simulink model "IEEE30_case"  (R2024b)
settings: Solver=FixedStepAuto  StartTime=0  StopTime=5  FixedStep=1e-7  RelTol=1e-3
values from neighbouring files (symbols this model uses):
  GFL_DFIG_7_C_bus = 0.08    [IEEE30_case_parameters.m]
  GFL_DFIG_7_D_mutual = 2.500000e+3    (= 2500)    [IEEE30_case_parameters.m]
  GFL_DFIG_7_f0 = 60    [IEEE30_case_parameters.m]
  GFL_DFIG_7_gPLLi = 3200    [IEEE30_case_parameters.m]
  GFL_DFIG_7_gPLLp = 650    [IEEE30_case_parameters.m]
  GFL_DFIG_7_H_WT = 0.4    [IEEE30_case_parameters.m]
  GFL_DFIG_7_Hg = 0.8    [IEEE30_case_parameters.m]
  GFL_DFIG_7_Igq_ref = 0    [IEEE30_case_parameters.m]
  GFL_DFIG_7_Ird_ref = 704.45696    [IEEE30_case_parameters.m]
  GFL_DFIG_7_KI_V = -300000    [IEEE30_case_parameters.m]
  GFL_DFIG_7_KP_V = -1000    [IEEE30_case_parameters.m]
  GFL_DFIG_7_Ksh = 1.254300e+4    (= 12543)    [IEEE30_case_parameters.m]
  GFL_DFIG_7_Lg = 0.000483    [IEEE30_case_parameters.m]
  GFL_DFIG_7_Lm_pu = 4    [IEEE30_case_parameters.m]
  GFL_DFIG_7_N = 100    [IEEE30_case_parameters.m]
  GFL_DFIG_7_p = 2    [IEEE30_case_parameters.m]
  GFL_DFIG_7_Pitch = 0    [IEEE30_case_parameters.m]
  GFL_DFIG_7_R = 44    [IEEE30_case_parameters.m]
  GFL_DFIG_7_Rg = 2.000000e-5    (= 2e-05)    [IEEE30_case_parameters.m]
  GFL_DFIG_7_rho = 1.225    [IEEE30_case_parameters.m]
  GFL_DFIG_7_rPLLi = 4500    [IEEE30_case_parameters.m]
  GFL_DFIG_7_rPLLp = 620    [IEEE30_case_parameters.m]
  GFL_DFIG_7_Rs_pu = 0.011    [IEEE30_case_parameters.m]
  GFL_DFIG_7_Sbase = 2.000000e+6    (= 2000000)    [IEEE30_case_parameters.m]
  GFL_DFIG_7_ugq_ref = 0    [IEEE30_case_parameters.m]
  GFL_DFIG_7_usd_ref = 0    [IEEE30_case_parameters.m]
  GFL_DFIG_7_Vbase = 690    [IEEE30_case_parameters.m]
  GFL_DFIG_7_Vdc_ref = 1200    [IEEE30_case_parameters.m]
  GFL_DFIG_7_wind = 12    [IEEE30_case_parameters.m]
  GFL_DFIG_7_wm_ref = 518.184209    [IEEE30_case_parameters.m]
  SG_D_13_D = 0.01056    [IEEE30_case_parameters.m]
  SG_D_13_EnableSaturation = 0    [IEEE30_case_parameters.m]
  SG_D_13_f0 = 60    [IEEE30_case_parameters.m]
  SG_D_13_H = 7.5    [IEEE30_case_parameters.m]
  SG_D_13_K_A = 20    [IEEE30_case_parameters.m]
  SG_D_13_K_E = 1.000000e+1    (= 10)    [IEEE30_case_parameters.m]
  SG_D_13_K_F = 2.363    [IEEE30_case_parameters.m]
  SG_D_13_K_s = 0.5    [IEEE30_case_parameters.m]
  SG_D_13_R_a = 0.001088    [IEEE30_case_parameters.m]
  SG_D_13_S_A = 1    [IEEE30_case_parameters.m]
  SG_D_13_S_B = 0.103    [IEEE30_case_parameters.m]
  SG_D_13_S_N = 10.659857    [IEEE30_case_parameters.m]
  SG_D_13_SpeedPara = 200    [IEEE30_case_parameters.m]
  SG_D_13_T_0 = 0.370163    [IEEE30_case_parameters.m]
  SG_D_13_T_1 = 0.3    [IEEE30_case_parameters.m]
  SG_D_13_T_2 = 0.05    [IEEE30_case_parameters.m]
  SG_D_13_T_3 = 0.02    [IEEE30_case_parameters.m]
  SG_D_13_T_4 = 0.005    [IEEE30_case_parameters.m]
  SG_D_13_T_A = 0.02    [IEEE30_case_parameters.m]
  SG_D_13_T_dd = 8.000000e+0    (= 8)    [IEEE30_case_parameters.m]
  SG_D_13_T_ddd = 0.04    [IEEE30_case_parameters.m]
  SG_D_13_T_E = 0.314    [IEEE30_case_parameters.m]
  SG_D_13_T_F = 0.35    [IEEE30_case_parameters.m]
  SG_D_13_T_qd = 0.8    [IEEE30_case_parameters.m]
  SG_D_13_T_qdd = 0.02    [IEEE30_case_parameters.m]
  SG_D_13_T_speed = 0.1    [IEEE30_case_parameters.m]
  SG_D_13_T_w = 0.5    [IEEE30_case_parameters.m]
  SG_D_13_V_ref = 1.696619    [IEEE30_case_parameters.m]
  SG_D_13_w_ref = 376.991118    [IEEE30_case_parameters.m]
  SG_D_13_x_d = 1.9    [IEEE30_case_parameters.m]
  SG_D_13_x_dd = 0.302    [IEEE30_case_parameters.m]
  SG_D_13_x_ddd = 0.204    [IEEE30_case_parameters.m]
  SG_D_13_x_l = 0.05    [IEEE30_case_parameters.m]
  SG_D_13_x_q = 1.3    [IEEE30_case_parameters.m]
  SG_D_13_x_qd = 0.5    [IEEE30_case_parameters.m]
  SG_D_13_x_qdd = 0.3    [IEEE30_case_parameters.m]
  SG_D_1_D = 0.01056    [IEEE30_case_parameters.m]
  SG_D_1_EnableSaturation = 0    [IEEE30_case_parameters.m]
  SG_D_1_f0 = 60    [IEEE30_case_parameters.m]
  SG_D_1_H = 7.5    [IEEE30_case_parameters.m]
  SG_D_1_K_A = 20    [IEEE30_case_parameters.m]
  SG_D_1_K_E = 1.000000e+1    (= 10)    [IEEE30_case_parameters.m]
  SG_D_1_K_F = 2.363    [IEEE30_case_parameters.m]
  SG_D_1_K_s = 0.5    [IEEE30_case_parameters.m]
  SG_D_1_R_a = 0.001088    [IEEE30_case_parameters.m]
  SG_D_1_S_A = 1    [IEEE30_case_parameters.m]
  SG_D_1_S_B = 0.103    [IEEE30_case_parameters.m]
  SG_D_1_S_N = 10.659857    [IEEE30_case_parameters.m]
  SG_D_1_SpeedPara = 200    [IEEE30_case_parameters.m]
  SG_D_1_T_0 = 0.259812    [IEEE30_case_parameters.m]
  SG_D_1_T_1 = 0.3    [IEEE30_case_parameters.m]
  SG_D_1_T_2 = 0.05    [IEEE30_case_parameters.m]
  SG_D_1_T_3 = 0.02    [IEEE30_case_parameters.m]
  SG_D_1_T_4 = 0.005    [IEEE30_case_parameters.m]
  SG_D_1_T_A = 0.02    [IEEE30_case_parameters.m]
  SG_D_1_T_dd = 8.000000e+0    (= 8)    [IEEE30_case_parameters.m]
  SG_D_1_T_ddd = 0.04    [IEEE30_case_parameters.m]
  SG_D_1_T_E = 0.314    [IEEE30_case_parameters.m]
  SG_D_1_T_F = 0.35    [IEEE30_case_parameters.m]
  SG_D_1_T_qd = 0.8    [IEEE30_case_parameters.m]
  SG_D_1_T_qdd = 0.02    [IEEE30_case_parameters.m]
  SG_D_1_T_speed = 0.1    [IEEE30_case_parameters.m]
  SG_D_1_T_w = 0.5    [IEEE30_case_parameters.m]
  SG_D_1_V_ref = 1.544107    [IEEE30_case_parameters.m]
  SG_D_1_w_ref = 376.991118    [IEEE30_case_parameters.m]
  SG_D_1_x_d = 1.9    [IEEE30_case_parameters.m]
  SG_D_1_x_dd = 0.302    [IEEE30_case_parameters.m]
  SG_D_1_x_ddd = 0.204    [IEEE30_case_parameters.m]
  SG_D_1_x_l = 0.05    [IEEE30_case_parameters.m]
  SG_D_1_x_q = 1.3    [IEEE30_case_parameters.m]
  SG_D_1_x_qd = 0.5    [IEEE30_case_parameters.m]
  SG_D_1_x_qdd = 0.3    [IEEE30_case_parameters.m]
  SG_D_22_D = 0.01056    [IEEE30_case_parameters.m]
  SG_D_22_EnableSaturation = 0    [IEEE30_case_parameters.m]
  SG_D_22_f0 = 60    [IEEE30_case_parameters.m]
  SG_D_22_H = 7.5    [IEEE30_case_parameters.m]
  SG_D_22_K_A = 20    [IEEE30_case_parameters.m]
  SG_D_22_K_E = 1.000000e+1    (= 10)    [IEEE30_case_parameters.m]
  SG_D_22_K_F = 2.363    [IEEE30_case_parameters.m]
  SG_D_22_K_s = 0.5    [IEEE30_case_parameters.m]
  SG_D_22_R_a = 0.001088    [IEEE30_case_parameters.m]
  SG_D_22_S_A = 1    [IEEE30_case_parameters.m]
  SG_D_22_S_B = 0.103    [IEEE30_case_parameters.m]
  SG_D_22_S_N = 10.659857    [IEEE30_case_parameters.m]
  SG_D_22_SpeedPara = 200    [IEEE30_case_parameters.m]
  SG_D_22_T_0 = 0.216121    [IEEE30_case_parameters.m]
  SG_D_22_T_1 = 0.3    [IEEE30_case_parameters.m]
  SG_D_22_T_2 = 0.05    [IEEE30_case_parameters.m]
  SG_D_22_T_3 = 0.02    [IEEE30_case_parameters.m]
  SG_D_22_T_4 = 0.005    [IEEE30_case_parameters.m]
  ... (+126 more)
(part 26 of 27)

== system IEEE30_case/SG_D_27/d_V_f_SG_D_27_block ==
  note: d_V_f_SG_D_27 in IEEE30_case
      | $-\frac{V_{f,\mathrm{SG},D,27}-K_{A}\,\left(V_{\mathrm{ref}}-\sqrt{{\left(\frac{R_{a}\,\left(\frac{\psi _{\mathrm{1d},\mathrm{SG},D,27}\,\left(x_{\mathrm{dd}}-x_{\mathrm{ddd}}\right)}{x_{\mathrm{dd}}-x_{l}}-\psi _{d,\mathrm{SG},D,27}+\frac{\psi _{\mathrm{fd},\mathrm{SG},D,27}\,\left(x_{\mathrm{ddd}}-x_{l}\right)}{x_{\mathrm{dd}}-x_{l}}\right)}{x_{\mathrm{ddd}}}+\frac{\psi _{q,\mathrm{SG},D,27}\,w_{\mathrm{SG},D,27}}{2\,f_{0}\,\pi }\right)}^2+{\left(\frac{R_{a}\,\left(\psi _{q,\mathrm{SG},D,27}+\frac{\psi _{\mathrm{gq},\mathrm{SG},D,27}\,\left(x_{l}-x_{\mathrm{qdd}}\right)}{x_{l}-x_{\mathrm{qd}}}+\frac{\psi _{\mathrm{kq},\mathrm{SG},D,27}\,\left(x_{\mathrm{qd}}-x_{\mathrm{qdd}}\right)}{x_{l}-x_{\mathrm{qd}}}\right)}{x_{\mathrm{qdd}}}+\frac{\psi _{d,\mathrm{SG},D,27}\,w_{\mathrm{SG},D,27}}{2\,f_{0}\,\pi }\right)}^2}+K_{s}\,\mathrm{Px}_{3,\mathrm{SG},D,27}\right)-K_{A}\,R_{f,\mathrm{SG},D,27}+\frac{E_{\mathrm{fd},\mathrm{SG},D,27}\,K_{A}\,K_{F}}{T_{F}}}{T_{A}}$
      | Automatically generated on 2025-11-01 18:38:43 .
  State_E_fd_SG_D_27_11911 : Inport
  State_R_f_SG_D_27_2a887 : Inport  Port=2
  State_Px_3_SG_D_27_cca99 : Inport  Port=3
  State_psi_1d_SG_D_27_082ae : Inport  Port=4
  State_psi_d_SG_D_27_7c091 : Inport  Port=5
  State_psi_fd_SG_D_27_27c3c : Inport  Port=6
  State_psi_q_SG_D_27_dd61c : Inport  Port=7
  State_w_SG_D_27_ac390 : Inport  Port=8
  State_psi_gq_SG_D_27_6c126 : Inport  Port=9
  State_psi_kq_SG_D_27_28d7a : Inport  Port=10
  State_psi_q_SG_D_27_7ebac : Inport  Port=11
  State_psi_d_SG_D_27_c8afe : Inport  Port=12
  State_w_SG_D_27_f905c : Inport  Port=13
  State_V_f_SG_D_27_03782 : Inport  Port=14
  Add_0078a : Sum
  Add_11ebf : Sum
  Add_49114 : Sum
  Add_7f7d3 : Sum
  Add_94690 : Sum
  Add_95553 : Sum
  Add_a6206 : Sum
  Add_c1965 : Sum
  Add_cb711 : Sum
  Add_ec3d2 : Sum
  Add_fc045 : Sum
  Constant_-1_000a4 : Constant  Value=-1
  Constant_-1_049db : Constant  Value=-1
  Constant_-1_8f4b4 : Constant  Value=-1
  Constant_-1_d241f : Constant  Value=-1
  Constant_-1_dbd36 : Constant  Value=-1
  Constant_-1_dc108 : Constant  Value=-1
  Constant_2.0_3de53 : Constant  Value=2.0
  Constant_2.0_7e780 : Constant  Value=2.0
  Constant_2.0_cb466 : Constant  Value=2.0
  Constant_2.0_f5381 : Constant  Value=2.0
  Constant_K_A_68bea : Constant  Value=K_A
  Constant_K_A_bb3c1 : Constant  Value=K_A
  Constant_K_A_fd187 : Constant  Value=K_A
  Constant_K_F_7b9a8 : Constant  Value=K_F
  Constant_K_s_9c7f8 : Constant  Value=K_s
  Constant_R_a_99a15 : Constant  Value=R_a
  Constant_R_a_d0966 : Constant  Value=R_a
  Constant_T_A_b480d : Constant  Value=T_A
  Constant_T_F_69b79 : Constant  Value=T_F
  Constant_V_ref_b0cb6 : Constant  Value=V_ref
  Constant_f0_2b603 : Constant  Value=f0
  Constant_f0_d9137 : Constant  Value=f0
  Constant_pi_56945 : Constant  Value=pi
  Constant_pi_ffc0e : Constant  Value=pi
  Constant_x_dd_a9468 : Constant  Value=x_dd
  Constant_x_dd_b4216 : Constant  Value=x_dd
  Constant_x_dd_f5ebf : Constant  Value=x_dd
  Constant_x_ddd_02d42 : Constant  Value=x_ddd
  Constant_x_ddd_4227a : Constant  Value=x_ddd
  Constant_x_ddd_9297d : Constant  Value=x_ddd
  Constant_x_l_3070b : Constant  Value=x_l
  Constant_x_l_69625 : Constant  Value=x_l
  Constant_x_l_6af3f : Constant  Value=x_l
  Constant_x_l_6fbfe : Constant  Value=x_l
  Constant_x_l_b5281 : Constant  Value=x_l
  Constant_x_l_cfd51 : Constant  Value=x_l
  Constant_x_qd_26019 : Constant  Value=x_qd
  Constant_x_qd_2f63a : Constant  Value=x_qd
  Constant_x_qd_be1f0 : Constant  Value=x_qd
  Constant_x_qdd_5a1b7 : Constant  Value=x_qdd
  Constant_x_qdd_794bf : Constant  Value=x_qdd
  Constant_x_qdd_96938 : Constant  Value=x_qdd
  Divide_07c87 : Product  Inputs=*/
  Divide_1f6ef : Product  Inputs=*/
  Divide_445bd : Product  Inputs=*/
  Divide_51106 : Product  Inputs=*/
  Divide_60db4 : Product  Inputs=*/
  Divide_9589b : Product  Inputs=*/
  Divide_b7d65 : Product  Inputs=*/
  Divide_c1438 : Product  Inputs=*/
  Divide_ee8b4 : Product  Inputs=*/
  Divide_f9c68 : Product  Inputs=*/
  MathFunc_sqrt_eec58 : Sqrt
  Power_7f54e : Math  Operator=pow
  Power_84ab0 : Math  Operator=pow
  Product_09536 : Product
  Product_0e0d1 : Product
  Product_13110 : Product
  Product_152fc : Product
  Product_226c9 : Product
  Product_24809 : Product
  Product_2dce1 : Product
  Product_374ff : Product
  Product_3d675 : Product
  Product_4e57c : Product
  Product_4e8b3 : Product
  Product_6396f : Product
  Product_6fef3 : Product
  Product_9a636 : Product
  Product_9b4d0 : Product
  Product_9db0a : Product
  Product_a1a64 : Product
  Product_bfec4 : Product
  Product_c6a00 : Product
  Product_d307f : Product
  Product_d8d42 : Product
  Product_dc7be : Product
  Product_f2389 : Product
  Subtract_0c442 : Sum  Inputs=+-
  Subtract_134c1 : Sum  Inputs=+-
  Subtract_192bb : Sum  Inputs=+-
  Subtract_29f06 : Sum  Inputs=+-
  Subtract_5e59d : Sum  Inputs=+-
  Subtract_5eac6 : Sum  Inputs=+-
  Subtract_680e4 : Sum  Inputs=+-
  Subtract_9d8d6 : Sum  Inputs=+-
  Subtract_cad22 : Sum  Inputs=+-
  Blockout_d_V_f_SG_D_27_ad652 : Outport
  wires:
  Constant_-1_049db/1 -> Product_374ff/1
  Constant_x_qdd_96938/1 -> Add_7f7d3/2
  Subtract_0c442/1 -> Product_09536/2
  State_psi_d_SG_D_27_c8afe/1 -> Product_bfec4/1
  Constant_x_ddd_9297d/1 -> Subtract_0c442/2
  Constant_f0_d9137/1 -> Product_9a636/2
  Constant_-1_dbd36/1 -> Product_6396f/1
  Constant_pi_ffc0e/1 -> Product_9b4d0/2
  Product_6396f/1 -> Add_7f7d3/1
  Product_374ff/1 -> Add_11ebf/1
  Product_6fef3/1 -> Product_226c9/1
  Constant_x_l_cfd51/1 -> Product_6396f/2
  Constant_-1_8f4b4/1 -> Product_6fef3/1
  Constant_-1_000a4/1 -> Product_0e0d1/1
  State_psi_1d_SG_D_27_082ae/1 -> Product_0e0d1/2
  Constant_x_dd_a9468/1 -> Subtract_0c442/1
  Constant_-1_dc108/1 -> Product_a1a64/1
  Constant_x_qd_be1f0/1 -> Subtract_5e59d/1
  Constant_x_l_6af3f/1 -> Product_a1a64/2
  Add_a6206/1 -> Divide_1f6ef/2
  Constant_x_qdd_794bf/1 -> Subtract_5e59d/2
  Constant_x_l_6fbfe/1 -> Product_374ff/2
  Product_0e0d1/1 -> Product_09536/1
  Constant_2.0_f5381/1 -> Product_c6a00/1
  Constant_x_dd_f5ebf/1 -> Subtract_9d8d6/1
  Constant_pi_56945/1 -> Product_c6a00/2
  Divide_07c87/1 -> Add_fc045/1
  Constant_x_l_3070b/1 -> Subtract_9d8d6/2
  State_w_SG_D_27_ac390/1 -> Product_4e57c/2
  Subtract_192bb/1 -> Product_9db0a/2
  Constant_x_ddd_4227a/1 -> Subtract_192bb/1
  Constant_x_l_69625/1 -> Subtract_192bb/2
  State_psi_gq_SG_D_27_6c126/1 -> Product_24809/1
  Add_7f7d3/1 -> Product_24809/2
  Product_a1a64/1 -> Add_a6206/1
  MathFunc_sqrt_eec58/1 -> Subtract_680e4/2
  Product_2dce1/1 -> Divide_b7d65/1
  Constant_x_qd_2f63a/1 -> Add_a6206/2
  State_psi_kq_SG_D_27_28d7a/1 -> Product_2dce1/1
  Subtract_5e59d/1 -> Product_2dce1/2
  Divide_51106/1 -> Subtract_134c1/2
  Constant_x_qd_26019/1 -> Add_11ebf/2
  State_psi_d_SG_D_27_7c091/1 -> Add_fc045/2
  Product_09536/1 -> Divide_07c87/1
  Subtract_9d8d6/1 -> Divide_07c87/2
  Product_9db0a/1 -> Divide_51106/1
  State_psi_fd_SG_D_27_27c3c/1 -> Product_9db0a/1
  Subtract_cad22/1 -> Divide_51106/2
  Constant_x_dd_b4216/1 -> Subtract_cad22/1
  Constant_x_l_b5281/1 -> Subtract_cad22/2
  Product_24809/1 -> Divide_1f6ef/1
  Product_226c9/1 -> Divide_9589b/1
  Add_11ebf/1 -> Divide_b7d65/2
  Divide_1f6ef/1 -> Subtract_5eac6/1
  Divide_b7d65/1 -> Subtract_5eac6/2
  Constant_R_a_d0966/1 -> Product_6fef3/2
  Add_fc045/1 -> Subtract_134c1/1
  Constant_2.0_cb466/1 -> Product_9b4d0/1
  Subtract_5eac6/1 -> Add_49114/1
  State_psi_q_SG_D_27_7ebac/1 -> Add_49114/2
  Subtract_134c1/1 -> Product_226c9/2
  State_psi_q_SG_D_27_dd61c/1 -> Product_4e57c/1
  Product_9b4d0/1 -> Product_9a636/1
  Constant_R_a_99a15/1 -> Product_13110/1
  Add_49114/1 -> Product_13110/2
  State_w_SG_D_27_f905c/1 -> Product_bfec4/2
  Product_c6a00/1 -> Product_152fc/1
  Constant_f0_2b603/1 -> Product_152fc/2
  Constant_x_ddd_02d42/1 -> Divide_9589b/2
  Product_4e57c/1 -> Divide_60db4/1
  Product_9a636/1 -> Divide_60db4/2
  Constant_-1_d241f/1 -> Product_d307f/1
  Product_13110/1 -> Divide_f9c68/1
  Constant_x_qdd_5a1b7/1 -> Divide_f9c68/2
  Product_bfec4/1 -> Divide_445bd/1
  Product_152fc/1 -> Divide_445bd/2
  Divide_9589b/1 -> Add_94690/1
  Divide_60db4/1 -> Add_94690/2
  Divide_f9c68/1 -> Add_0078a/1
  Divide_445bd/1 -> Add_0078a/2
  State_E_fd_SG_D_27_11911/1 -> Product_d307f/2
  Add_94690/1 -> Power_7f54e/1
  Constant_2.0_7e780/1 -> Power_7f54e/2
  Add_0078a/1 -> Power_84ab0/1
  Constant_2.0_3de53/1 -> Power_84ab0/2
  Product_d307f/1 -> Product_d8d42/1
  Constant_K_A_bb3c1/1 -> Product_d8d42/2
  Constant_K_s_9c7f8/1 -> Product_dc7be/1
  State_Px_3_SG_D_27_cca99/1 -> Product_dc7be/2
  Power_7f54e/1 -> Add_cb711/1
  Power_84ab0/1 -> Add_cb711/2
  Product_d8d42/1 -> Product_f2389/1
  Constant_K_F_7b9a8/1 -> Product_f2389/2
  Product_dc7be/1 -> Add_ec3d2/1
  Constant_V_ref_b0cb6/1 -> Add_ec3d2/2
  Add_cb711/1 -> MathFunc_sqrt_eec58/1
  Product_f2389/1 -> Divide_c1438/1
  Constant_T_F_69b79/1 -> Divide_c1438/2
  Constant_K_A_68bea/1 -> Product_4e8b3/1
  State_R_f_SG_D_27_2a887/1 -> Product_4e8b3/2
  Add_ec3d2/1 -> Subtract_680e4/1
  Divide_c1438/1 -> Add_95553/1
  Product_4e8b3/1 -> Add_95553/2
  Constant_K_A_fd187/1 -> Product_3d675/1
  Subtract_680e4/1 -> Product_3d675/2
  Add_95553/1 -> Add_c1965/1
  Product_3d675/1 -> Add_c1965/2
  Add_c1965/1 -> Subtract_29f06/1
  State_V_f_SG_D_27_03782/1 -> Subtract_29f06/2
  Subtract_29f06/1 -> Divide_ee8b4/1
  Constant_T_A_b480d/1 -> Divide_ee8b4/2
  Divide_ee8b4/1 -> Blockout_d_V_f_SG_D_27_ad652/1

== system IEEE30_case/SG_D_27/d_psi_1d_SG_D_27_block ==
  note: d_psi_1d_SG_D_27 in IEEE30_case
      | $-\frac{\psi _{\mathrm{1d},\mathrm{SG},D,27}-\psi _{\mathrm{fd},\mathrm{SG},D,27}+\frac{\left(x_{\mathrm{dd}}-x_{l}\right)\,\left(\frac{\psi _{\mathrm{1d},\mathrm{SG},D,27}\,\left(x_{\mathrm{dd}}-x_{\mathrm{ddd}}\right)}{x_{\mathrm{dd}}-x_{l}}-\psi _{d,\mathrm{SG},D,27}+\frac{\psi _{\mathrm{fd},\mathrm{SG},D,27}\,\left(x_{\mathrm{ddd}}-x_{l}\right)}{x_{\mathrm{dd}}-x_{l}}\right)}{x_{\mathrm{ddd}}}}{T_{\mathrm{ddd}}}$
      | Automatically generated on 2025-11-01 18:38:18 .
  State_psi_1d_SG_D_27_efe98 : Inport
  State_psi_fd_SG_D_27_72b20 : Inport  Port=2
  State_psi_1d_SG_D_27_d0b37 : Inport  Port=3
  State_psi_d_SG_D_27_a8139 : Inport  Port=4
  State_psi_fd_SG_D_27_15400 : Inport  Port=5
  Add_984ac : Sum
  Add_acd11 : Sum
  Add_e0ec5 : Sum
  Constant_-1_6684c : Constant  Value=-1
  Constant_-1_d4480 : Constant  Value=-1
  Constant_T_ddd_242a5 : Constant  Value=T_ddd
  Constant_x_dd_17d37 : Constant  Value=x_dd
  Constant_x_dd_9a35f : Constant  Value=x_dd
  Constant_x_dd_b2bbb : Constant  Value=x_dd
  Constant_x_dd_dacc0 : Constant  Value=x_dd
  Constant_x_ddd_1b643 : Constant  Value=x_ddd
  Constant_x_ddd_29fd3 : Constant  Value=x_ddd
  Constant_x_ddd_4cc24 : Constant  Value=x_ddd
  Constant_x_l_274a7 : Constant  Value=x_l
  Constant_x_l_7e31f : Constant  Value=x_l
  Constant_x_l_91910 : Constant  Value=x_l
  Constant_x_l_d8697 : Constant  Value=x_l
  Divide_285f2 : Product  Inputs=*/
  Divide_554ff : Product  Inputs=*/
  Divide_6beb7 : Product  Inputs=*/
  Divide_8ca94 : Product  Inputs=*/
  Product_3b738 : Product
  Product_6cf61 : Product
  Product_94cdb : Product
  Product_b5c9b : Product
  Product_e0e6d : Product
  Subtract_5443c : Sum  Inputs=+-
  Subtract_b034b : Sum  Inputs=+-
  Subtract_ca0ec : Sum  Inputs=+-
  Subtract_d97b4 : Sum  Inputs=+-
  Subtract_f1971 : Sum  Inputs=+-
  Subtract_fd591 : Sum  Inputs=+-
  Blockout_d_psi_1d_SG_D_27_6915f : Outport
  wires:
  Constant_-1_6684c/1 -> Product_e0e6d/1
  State_psi_1d_SG_D_27_d0b37/1 -> Product_e0e6d/2
  Subtract_ca0ec/1 -> Product_6cf61/2
  Constant_x_ddd_1b643/1 -> Subtract_ca0ec/1
  Constant_x_dd_9a35f/1 -> Subtract_5443c/1
  Product_e0e6d/1 -> Product_b5c9b/1
  Subtract_f1971/1 -> Product_3b738/1
  Constant_x_dd_dacc0/1 -> Subtract_d97b4/1
  Constant_x_ddd_4cc24/1 -> Subtract_5443c/2
  Add_e0ec5/1 -> Add_acd11/1
  Subtract_5443c/1 -> Product_b5c9b/2
  Constant_x_l_274a7/1 -> Subtract_d97b4/2
  Add_acd11/1 -> Divide_8ca94/1
  Constant_x_l_7e31f/1 -> Subtract_ca0ec/2
  Product_b5c9b/1 -> Divide_554ff/1
  Subtract_d97b4/1 -> Divide_554ff/2
  Product_6cf61/1 -> Divide_285f2/1
  State_psi_fd_SG_D_27_15400/1 -> Product_6cf61/1
  Subtract_fd591/1 -> Divide_285f2/2
  Constant_x_dd_17d37/1 -> Subtract_fd591/1
  Constant_x_l_91910/1 -> Subtract_fd591/2
  Divide_554ff/1 -> Add_984ac/1
  Divide_285f2/1 -> Subtract_b034b/2
  State_psi_d_SG_D_27_a8139/1 -> Add_984ac/2
  Constant_x_dd_b2bbb/1 -> Subtract_f1971/1
  Constant_x_l_d8697/1 -> Subtract_f1971/2
  Add_984ac/1 -> Subtract_b034b/1
  Constant_-1_d4480/1 -> Product_94cdb/1
  State_psi_1d_SG_D_27_efe98/1 -> Product_94cdb/2
  Subtract_b034b/1 -> Product_3b738/2
  Product_94cdb/1 -> Add_e0ec5/1
  Product_3b738/1 -> Divide_6beb7/1
  State_psi_fd_SG_D_27_72b20/1 -> Add_e0ec5/2
  Constant_x_ddd_29fd3/1 -> Divide_6beb7/2
  Divide_6beb7/1 -> Add_acd11/2
  Constant_T_ddd_242a5/1 -> Divide_8ca94/2
  Divide_8ca94/1 -> Blockout_d_psi_1d_SG_D_27_6915f/1

== system IEEE30_case/SG_D_27/d_psi_d_SG_D_27_block ==
  note: d_psi_d_SG_D_27 in IEEE30_case
      | $2\,\pi \,f_{0}\,\left(v_{d,\mathrm{SG},D,27}\,\sin\left(\theta _{\mathrm{SG},D,27}\right)-v_{q,\mathrm{SG},D,27}\,\cos\left(\theta _{\mathrm{SG},D,27}\right)+\frac{R_{a}\,\left(\frac{\psi _{\mathrm{1d},\mathrm{SG},D,27}\,\left(x_{\mathrm{dd}}-x_{\mathrm{ddd}}\right)}{x_{\mathrm{dd}}-x_{l}}-\psi _{d,\mathrm{SG},D,27}+\frac{\psi _{\mathrm{fd},\mathrm{SG},D,27}\,\left(x_{\mathrm{ddd}}-x_{l}\right)}{x_{\mathrm{dd}}-x_{l}}\right)}{x_{\mathrm{ddd}}}+\frac{\psi _{q,\mathrm{SG},D,27}\,w_{\mathrm{SG},D,27}}{2\,f_{0}\,\pi }\right)$
      | Automatically generated on 2025-11-01 18:38:06 .
  State_psi_1d_SG_D_27_d5c1b : Inport
  State_psi_d_SG_D_27_a7f1f : Inport  Port=2
  State_psi_fd_SG_D_27_62224 : Inport  Port=3
  Input_v_d_SG_D_27_222f7 : Inport  Port=4
  State_theta_SG_D_27_17b48 : Inport  Port=5
  Input_v_q_SG_D_27_3207e : Inport  Port=6
  State_theta_SG_D_27_9f539 : Inport  Port=7
  State_psi_q_SG_D_27_a07c2 : Inport  Port=8
  State_w_SG_D_27_e9387 : Inport  Port=9
  Add_d6796 : Sum
  Add_dd900 : Sum
  Constant_-1_cafcc : Constant  Value=-1
  Constant_-2.0_1580e : Constant  Value=-2.0
  Constant_2.0_b6be6 : Constant  Value=2.0
  Constant_R_a_4194c : Constant  Value=R_a
  Constant_f0_77b52 : Constant  Value=f0
  Constant_f0_a4d71 : Constant  Value=f0
  Constant_pi_01718 : Constant  Value=pi
  Constant_pi_76666 : Constant  Value=pi
  Constant_x_dd_97fe1 : Constant  Value=x_dd
  Constant_x_dd_b2359 : Constant  Value=x_dd
  Constant_x_dd_c11b2 : Constant  Value=x_dd
  Constant_x_ddd_27033 : Constant  Value=x_ddd
  Constant_x_ddd_5a17f : Constant  Value=x_ddd
  Constant_x_ddd_f3053 : Constant  Value=x_ddd
  Constant_x_l_15a75 : Constant  Value=x_l
  Constant_x_l_b602a : Constant  Value=x_l
  Constant_x_l_bf8de : Constant  Value=x_l
  Divide_39e1c : Product  Inputs=*/
  Divide_7b2f6 : Product  Inputs=*/
  Divide_87c62 : Product  Inputs=*/
  Divide_b4afa : Product  Inputs=*/
  MathFunc_cos_0d1ba : Trigonometry  Operator=cos
  MathFunc_sin_08222 : Trigonometry
  Product_08f41 : Product
  Product_26066 : Product
  Product_58d64 : Product
  Product_71de0 : Product
  Product_745cc : Product
  Product_8936f : Product
  Product_9d16b : Product
  Product_a21c8 : Product
  Product_c5893 : Product
  Product_ee8b1 : Product
  Product_f3a5d : Product
  Product_f47ea : Product
  Subtract_062b2 : Sum  Inputs=+-
  Subtract_1848d : Sum  Inputs=+-
  Subtract_3d9d4 : Sum  Inputs=+-
  Subtract_5c54f : Sum  Inputs=+-
  Subtract_5feb8 : Sum  Inputs=+-
  Subtract_ab593 : Sum  Inputs=+-
  Subtract_bcda1 : Sum  Inputs=+-
  Blockout_d_psi_d_SG_D_27_ed15c : Outport
  wires:
  Divide_b4afa/1 -> Subtract_1848d/1
  Constant_x_l_15a75/1 -> Subtract_5feb8/2
  Constant_-1_cafcc/1 -> Product_a21c8/1
  Constant_x_dd_b2359/1 -> Subtract_5feb8/1
  State_psi_1d_SG_D_27_d5c1b/1 -> Product_a21c8/2
  Constant_x_dd_c11b2/1 -> Subtract_bcda1/1
  Product_8936f/1 -> Divide_b4afa/1
  Constant_x_ddd_f3053/1 -> Subtract_bcda1/2
  Product_a21c8/1 -> Product_71de0/1
  Subtract_bcda1/1 -> Product_71de0/2
  Product_26066/1 -> Product_c5893/1
  State_w_SG_D_27_e9387/1 -> Product_745cc/2
  Constant_x_ddd_27033/1 -> Subtract_5c54f/1
  Constant_x_l_bf8de/1 -> Subtract_5c54f/2
  Product_71de0/1 -> Divide_39e1c/1
  Subtract_5feb8/1 -> Divide_39e1c/2
  State_psi_fd_SG_D_27_62224/1 -> Product_9d16b/1
  Subtract_5c54f/1 -> Product_9d16b/2
  Constant_x_dd_97fe1/1 -> Subtract_062b2/1
  State_theta_SG_D_27_9f539/1 -> MathFunc_cos_0d1ba/1
  Constant_x_l_b602a/1 -> Subtract_062b2/2
  Divide_39e1c/1 -> Add_dd900/1
  Add_d6796/1 -> Subtract_ab593/1
  State_psi_d_SG_D_27_a7f1f/1 -> Add_dd900/2
  Constant_f0_77b52/1 -> Product_26066/2
  Product_9d16b/1 -> Divide_7b2f6/1
  Subtract_062b2/1 -> Divide_7b2f6/2
  Add_dd900/1 -> Subtract_3d9d4/1
  Constant_pi_76666/1 -> Product_08f41/2
  Divide_7b2f6/1 -> Subtract_3d9d4/2
  Constant_R_a_4194c/1 -> Product_8936f/1
  Subtract_3d9d4/1 -> Product_8936f/2
  MathFunc_sin_08222/1 -> Product_f47ea/2
  State_theta_SG_D_27_17b48/1 -> MathFunc_sin_08222/1
  Constant_x_ddd_5a17f/1 -> Divide_b4afa/2
  Product_f47ea/1 -> Subtract_1848d/2
  Input_v_d_SG_D_27_222f7/1 -> Product_f47ea/1
  Constant_2.0_b6be6/1 -> Product_ee8b1/1
  Input_v_q_SG_D_27_3207e/1 -> Product_f3a5d/1
  Constant_pi_01718/1 -> Product_ee8b1/2
  Constant_f0_a4d71/1 -> Product_58d64/2
  MathFunc_cos_0d1ba/1 -> Product_f3a5d/2
  Product_745cc/1 -> Divide_87c62/1
  State_psi_q_SG_D_27_a07c2/1 -> Product_745cc/1
  Product_ee8b1/1 -> Product_58d64/1
  Product_08f41/1 -> Product_26066/1
  Constant_-2.0_1580e/1 -> Product_08f41/1
  Subtract_1848d/1 -> Add_d6796/1
  Product_c5893/1 -> Blockout_d_psi_d_SG_D_27_ed15c/1
  Product_f3a5d/1 -> Add_d6796/2
  Product_58d64/1 -> Divide_87c62/2
  Divide_87c62/1 -> Subtract_ab593/2
  Subtract_ab593/1 -> Product_c5893/2

== system IEEE30_case/SG_D_27/d_psi_fd_SG_D_27_block ==
  note: d_psi_fd_SG_D_27 in IEEE30_case
      | $-\frac{\psi _{\mathrm{fd},\mathrm{SG},D,27}-E_{\mathrm{fd},\mathrm{SG},D,27}+\left(x_{d}-x_{\mathrm{dd}}\right)\,\left(\frac{\frac{\psi _{\mathrm{1d},\mathrm{SG},D,27}\,\left(x_{\mathrm{dd}}-x_{\mathrm{ddd}}\right)}{x_{\mathrm{dd}}-x_{l}}-\psi _{d,\mathrm{SG},D,27}+\frac{\psi _{\mathrm{fd},\mathrm{SG},D,27}\,\left(x_{\mathrm{ddd}}-x_{l}\right)}{x_{\mathrm{dd}}-x_{l}}}{x_{\mathrm{ddd}}}-\frac{\left(x_{\mathrm{dd}}-x_{\mathrm{ddd}}\right)\,\left(\psi _{\mathrm{1d},\mathrm{SG},D,27}-\psi _{\mathrm{fd},\mathrm{SG},D,27}+\frac{\left(x_{\mathrm{dd}}-x_{l}\right)\,\left(\frac{\psi _{\mathrm{1d},\mathrm{SG},D,27}\,\left(x_{\mathrm{dd}}-x_{\mathrm{ddd}}\right)}{x_{\mathrm{dd}}-x_{l}}-\psi _{d,\mathrm{SG},D,27}+\frac{\psi _{\mathrm{fd},\mathrm{SG},D,27}\,\left(x_{\mathrm{ddd}}-x_{l}\right)}{x_{\mathrm{dd}}-x_{l}}\right)}{x_{\mathrm{ddd}}}\right)}{{\left(x_{\mathrm{dd}}-x_{l}\right)}^2}\right)}{T_{\mathrm{dd}}}$
      | Automatically generated on 2025-11-01 18:38:15 .
  State_E_fd_SG_D_27_fdb39 : Inport
  State_psi_fd_SG_D_27_68608 : Inport  Port=2
  State_psi_1d_SG_D_27_49a09 : Inport  Port=3
  State_psi_fd_SG_D_27_f02f4 : Inport  Port=4
  State_psi_1d_SG_D_27_946b5 : Inport  Port=5
  State_psi_d_SG_D_27_fdc2b : Inport  Port=6
  State_psi_fd_SG_D_27_a093b : Inport  Port=7
  State_psi_1d_SG_D_27_1e075 : Inport  Port=8
  State_psi_d_SG_D_27_0dbb0 : Inport  Port=9
  State_psi_fd_SG_D_27_a19a0 : Inport  Port=10
  Add_1e41a : Sum
  Add_bd06a : Sum
  Constant_-1_21ffa : Constant  Value=-1
  Constant_-1_63aa3 : Constant  Value=-1
  Constant_-1_e3612 : Constant  Value=-1
  Constant_2.0_818b3 : Constant  Value=2.0
  Constant_T_dd_bea5b : Constant  Value=T_dd
  Constant_x_d_3b58c : Constant  Value=x_d
  Constant_x_dd_09696 : Constant  Value=x_dd
  Constant_x_dd_1b1b4 : Constant  Value=x_dd
  Constant_x_dd_25c64 : Constant  Value=x_dd
  Constant_x_dd_2ff33 : Constant  Value=x_dd
  Constant_x_dd_4eee0 : Constant  Value=x_dd
  Constant_x_dd_872b1 : Constant  Value=x_dd
  Constant_x_dd_af76d : Constant  Value=x_dd
  Constant_x_dd_c3d0e : Constant  Value=x_dd
  Constant_x_dd_d30d3 : Constant  Value=x_dd
  Constant_x_dd_e6b63 : Constant  Value=x_dd
  Constant_x_ddd_564f0 : Constant  Value=x_ddd
  Constant_x_ddd_5d383 : Constant  Value=x_ddd
  Constant_x_ddd_661df : Constant  Value=x_ddd
  Constant_x_ddd_83567 : Constant  Value=x_ddd
  Constant_x_ddd_d2b11 : Constant  Value=x_ddd
  Constant_x_ddd_e02b5 : Constant  Value=x_ddd
  Constant_x_ddd_e5c8e : Constant  Value=x_ddd
  Constant_x_l_006dc : Constant  Value=x_l
  Constant_x_l_55923 : Constant  Value=x_l
  Constant_x_l_66cda : Constant  Value=x_l
  Constant_x_l_6f0a9 : Constant  Value=x_l
  Constant_x_l_885e3 : Constant  Value=x_l
  Constant_x_l_8f97e : Constant  Value=x_l
  Constant_x_l_e099f : Constant  Value=x_l
  Constant_x_l_f0ec2 : Constant  Value=x_l
  Divide_144f3 : Product  Inputs=*/
  Divide_1806d : Product  Inputs=*/
  Divide_429a5 : Product  Inputs=*/
  Divide_913bf : Product  Inputs=*/
  Divide_a4ff9 : Product  Inputs=*/
  Divide_d5a08 : Product  Inputs=*/
  Divide_d6d78 : Product  Inputs=*/
  Divide_f412e : Product  Inputs=*/
  Power_5d24d : Math  Operator=pow
  Product_227af : Product
  Product_3f658 : Product
  Product_4814e : Product
  Product_4a1e5 : Product
  Product_6b77f : Product
  Product_72f51 : Product
  Product_7e8bc : Product
  Product_e2615 : Product
  Product_f0d1b : Product
  Product_f7d09 : Product
  Subtract_02cec : Sum  Inputs=+-
  Subtract_2b2a0 : Sum  Inputs=+-
  Subtract_32fb0 : Sum  Inputs=+-
  Subtract_48462 : Sum  Inputs=+-
  Subtract_4f864 : Sum  Inputs=+-
  Subtract_5da30 : Sum  Inputs=+-
  Subtract_5e343 : Sum  Inputs=+-
  Subtract_627ab : Sum  Inputs=+-
  Subtract_62b0c : Sum  Inputs=+-
  Subtract_769bd : Sum  Inputs=+-
  Subtract_89f08 : Sum  Inputs=+-
  Subtract_b9389 : Sum  Inputs=+-
  Subtract_d5a6b : Sum  Inputs=+-
  Subtract_d63e6 : Sum  Inputs=+-
  Subtract_dade3 : Sum  Inputs=+-
  Subtract_e3e3d : Sum  Inputs=+-
  Subtract_e647a : Sum  Inputs=+-
  Subtract_eecd2 : Sum  Inputs=+-
  Subtract_f34b3 : Sum  Inputs=+-
  Blockout_d_psi_fd_SG_D_27_836bf : Outport
  wires:
  Constant_-1_21ffa/1 -> Product_72f51/1
  State_psi_1d_SG_D_27_946b5/1 -> Product_72f51/2
  Product_72f51/1 -> Product_f7d09/1
  Constant_x_dd_09696/1 -> Subtract_627ab/1
  Subtract_627ab/1 -> Product_f7d09/2
  Constant_x_ddd_d2b11/1 -> Subtract_627ab/2
  Constant_x_dd_e6b63/1 -> Subtract_dade3/1
  Subtract_d63e6/1 -> Product_6b77f/1
  Constant_x_dd_1b1b4/1 -> Subtract_d63e6/1
  Constant_x_l_006dc/1 -> Subtract_dade3/2
  Constant_x_ddd_e5c8e/1 -> Divide_429a5/2
  Subtract_e3e3d/1 -> Product_4814e/2
  Constant_x_ddd_564f0/1 -> Subtract_e3e3d/1
  Subtract_89f08/1 -> Divide_a4ff9/2
  Constant_x_dd_25c64/1 -> Subtract_89f08/1
  Constant_x_l_885e3/1 -> Subtract_e3e3d/2
  Product_f7d09/1 -> Divide_144f3/1
  Subtract_dade3/1 -> Divide_144f3/2
  Product_4814e/1 -> Divide_a4ff9/1
  State_psi_fd_SG_D_27_a093b/1 -> Product_4814e/1
  Constant_x_l_f0ec2/1 -> Subtract_89f08/2
  Divide_144f3/1 -> Add_bd06a/1
  Subtract_eecd2/1 -> Power_5d24d/1
  Constant_x_dd_c3d0e/1 -> Subtract_eecd2/1
  State_psi_d_SG_D_27_fdc2b/1 -> Add_bd06a/2
  Constant_x_l_66cda/1 -> Subtract_d63e6/2
  Add_bd06a/1 -> Subtract_32fb0/1
  Divide_a4ff9/1 -> Subtract_32fb0/2
  Product_e2615/1 -> Product_3f658/1
  Constant_-1_63aa3/1 -> Product_e2615/1
  Product_3f658/1 -> Divide_d5a08/1
  State_psi_1d_SG_D_27_1e075/1 -> Product_e2615/2
  Subtract_b9389/1 -> Product_3f658/2
  Constant_x_dd_872b1/1 -> Subtract_b9389/1
  Divide_d5a08/1 -> Add_1e41a/1
  Constant_x_ddd_e02b5/1 -> Subtract_b9389/2
  Subtract_32fb0/1 -> Product_6b77f/2
  Subtract_f34b3/1 -> Divide_d5a08/2
  Constant_x_dd_af76d/1 -> Subtract_f34b3/1
  Constant_x_l_6f0a9/1 -> Subtract_f34b3/2
  Constant_x_ddd_5d383/1 -> Divide_1806d/2
  Product_f0d1b/1 -> Product_7e8bc/1
  Subtract_62b0c/1 -> Product_4a1e5/2
  Constant_x_ddd_83567/1 -> Subtract_62b0c/1
  Subtract_02cec/1 -> Subtract_e647a/1
  Constant_x_l_55923/1 -> Subtract_62b0c/2
  Constant_x_dd_4eee0/1 -> Subtract_48462/1
  Subtract_d5a6b/1 -> Divide_d6d78/2
  Subtract_48462/1 -> Product_f0d1b/2
  Constant_x_dd_d30d3/1 -> Subtract_d5a6b/1
  Constant_x_ddd_661df/1 -> Subtract_48462/2
  State_psi_1d_SG_D_27_49a09/1 -> Subtract_02cec/1
  State_psi_fd_SG_D_27_f02f4/1 -> Subtract_02cec/2
  Product_6b77f/1 -> Divide_429a5/1
  Product_4a1e5/1 -> Divide_d6d78/1
  State_psi_fd_SG_D_27_a19a0/1 -> Product_4a1e5/1
  Constant_x_l_e099f/1 -> Subtract_d5a6b/2
  Constant_-1_e3612/1 -> Product_f0d1b/1
  Divide_429a5/1 -> Subtract_e647a/2
  Constant_x_l_8f97e/1 -> Subtract_eecd2/2
  State_psi_d_SG_D_27_0dbb0/1 -> Add_1e41a/2
  Subtract_e647a/1 -> Product_7e8bc/2
  Constant_2.0_818b3/1 -> Power_5d24d/2
  Add_1e41a/1 -> Subtract_769bd/1
  Divide_d6d78/1 -> Subtract_769bd/2
  Product_7e8bc/1 -> Divide_913bf/1
  Power_5d24d/1 -> Divide_913bf/2
  Subtract_769bd/1 -> Divide_1806d/1
  Constant_x_d_3b58c/1 -> Subtract_5da30/1
  Constant_x_dd_2ff33/1 -> Subtract_5da30/2
  Divide_913bf/1 -> Subtract_2b2a0/1
  Divide_1806d/1 -> Subtract_2b2a0/2
  State_E_fd_SG_D_27_fdb39/1 -> Subtract_5e343/1
  State_psi_fd_SG_D_27_68608/1 -> Subtract_5e343/2
  Subtract_5da30/1 -> Product_227af/1
  Subtract_2b2a0/1 -> Product_227af/2
  Subtract_5e343/1 -> Subtract_4f864/1
  Product_227af/1 -> Subtract_4f864/2
  Subtract_4f864/1 -> Divide_f412e/1
  Constant_T_dd_bea5b/1 -> Divide_f412e/2
  Divide_f412e/1 -> Blockout_d_psi_fd_SG_D_27_836bf/1

== system IEEE30_case/SG_D_27/d_psi_gq_SG_D_27_block ==
  note: d_psi_gq_SG_D_27 in IEEE30_case
      | $-\frac{\psi _{\mathrm{gq},\mathrm{SG},D,27}+\left(x_{q}-x_{\mathrm{qd}}\right)\,\left(\frac{\psi _{q,\mathrm{SG},D,27}+\frac{\psi _{\mathrm{gq},\mathrm{SG},D,27}\,\left(x_{l}-x_{\mathrm{qdd}}\right)}{x_{l}-x_{\mathrm{qd}}}+\frac{\psi _{\mathrm{kq},\mathrm{SG},D,27}\,\left(x_{\mathrm{qd}}-x_{\mathrm{qdd}}\right)}{x_{l}-x_{\mathrm{qd}}}}{x_{\mathrm{qdd}}}+\frac{\left(x_{\mathrm{qd}}-x_{\mathrm{qdd}}\right)\,\left(\psi _{\mathrm{gq},\mathrm{SG},D,27}+\psi _{\mathrm{kq},\mathrm{SG},D,27}+\frac{\left(x_{l}-x_{\mathrm{qd}}\right)\,\left(\psi _{q,\mathrm{SG},D,27}+\frac{\psi _{\mathrm{gq},\mathrm{SG},D,27}\,\left(x_{l}-x_{\mathrm{qdd}}\right)}{x_{l}-x_{\mathrm{qd}}}+\frac{\psi _{\mathrm{kq},\mathrm{SG},D,27}\,\left(x_{\mathrm{qd}}-x_{\mathrm{qdd}}\right)}{x_{l}-x_{\mathrm{qd}}}\right)}{x_{\mathrm{qdd}}}\right)}{{\left(x_{l}-x_{\mathrm{qd}}\right)}^2}\right)}{T_{\mathrm{qd}}}$
      | Automatically generated on 2025-11-01 18:38:24 .
  State_psi_gq_SG_D_27_c3af2 : Inport
  State_psi_gq_SG_D_27_6e8f7 : Inport  Port=2
  State_psi_kq_SG_D_27_7c836 : Inport  Port=3
  State_psi_gq_SG_D_27_3e2b9 : Inport  Port=4
  State_psi_kq_SG_D_27_4dbff : Inport  Port=5
  State_psi_q_SG_D_27_a0060 : Inport  Port=6
  State_psi_gq_SG_D_27_ed82f : Inport  Port=7
  State_psi_kq_SG_D_27_09d28 : Inport  Port=8
  State_psi_q_SG_D_27_f7919 : Inport  Port=9
  Add_1e70e : Sum
  Add_48da1 : Sum
  Add_4b738 : Sum
  Add_73542 : Sum
  Add_7e406 : Sum
  Add_85f35 : Sum
  Add_9c560 : Sum
  Add_b110a : Sum
  Add_bba7d : Sum
  Add_c43b7 : Sum
  Add_c9cb5 : Sum
  Add_e5e6a : Sum
  Constant_-1_058df : Constant  Value=-1
  Constant_-1_0983a : Constant  Value=-1
  Constant_-1_14dd2 : Constant  Value=-1
  Constant_-1_14efb : Constant  Value=-1
  Constant_-1_28226 : Constant  Value=-1
  Constant_-1_3ef3e : Constant  Value=-1
  Constant_-1_4fa86 : Constant  Value=-1
  Constant_-1_6b263 : Constant  Value=-1
  Constant_-1_9d686 : Constant  Value=-1
  Constant_-1_d0f9f : Constant  Value=-1
  Constant_2.0_312bc : Constant  Value=2.0
  Constant_T_qd_feea3 : Constant  Value=T_qd
  Constant_x_l_14cc6 : Constant  Value=x_l
  Constant_x_l_1677c : Constant  Value=x_l
  Constant_x_l_54f9f : Constant  Value=x_l
  Constant_x_l_793c4 : Constant  Value=x_l
  Constant_x_l_8c285 : Constant  Value=x_l
  Constant_x_l_a146c : Constant  Value=x_l
  Constant_x_l_d0309 : Constant  Value=x_l
  Constant_x_l_f9961 : Constant  Value=x_l
  Constant_x_q_90015 : Constant  Value=x_q
  Constant_x_qd_07190 : Constant  Value=x_qd
  Constant_x_qd_20e3c : Constant  Value=x_qd
  Constant_x_qd_38946 : Constant  Value=x_qd
  Constant_x_qd_5e3be : Constant  Value=x_qd
  Constant_x_qd_b0be0 : Constant  Value=x_qd
  Constant_x_qd_b7f1f : Constant  Value=x_qd
  Constant_x_qd_c908f : Constant  Value=x_qd
  Constant_x_qd_d4f0d : Constant  Value=x_qd
  Constant_x_qd_e9b47 : Constant  Value=x_qd
  Constant_x_qd_e9e12 : Constant  Value=x_qd
  Constant_x_qdd_51bb0 : Constant  Value=x_qdd
  Constant_x_qdd_699cd : Constant  Value=x_qdd
  Constant_x_qdd_6ad97 : Constant  Value=x_qdd
  Constant_x_qdd_81391 : Constant  Value=x_qdd
  Constant_x_qdd_bfc03 : Constant  Value=x_qdd
  Constant_x_qdd_e17ca : Constant  Value=x_qdd
  Constant_x_qdd_fe73c : Constant  Value=x_qdd
  Divide_2b076 : Product  Inputs=*/
  Divide_4a76a : Product  Inputs=*/
  Divide_638f3 : Product  Inputs=*/
  Divide_647d7 : Product  Inputs=*/
  Divide_a909f : Product  Inputs=*/
  Divide_b7c1d : Product  Inputs=*/
  Divide_cbeb0 : Product  Inputs=*/
  Divide_e205d : Product  Inputs=*/
  Power_6b5ce : Math  Operator=pow
  Product_1d788 : Product
  Product_242e9 : Product
  Product_26390 : Product
  Product_3603a : Product
  Product_450c3 : Product
  Product_56ad6 : Product
  Product_57164 : Product
  Product_8ca79 : Product
  Product_994b8 : Product
  Product_996e2 : Product
  Product_9be87 : Product
  Product_a6325 : Product
  Product_b10ae : Product
  Product_bef90 : Product
  Product_c8340 : Product
  Product_c97cd : Product
  Product_fec86 : Product
  Subtract_2a6c1 : Sum  Inputs=+-
  Subtract_3ad86 : Sum  Inputs=+-
  Subtract_808bf : Sum  Inputs=+-
  Subtract_84fe7 : Sum  Inputs=+-
  Subtract_a1eb2 : Sum  Inputs=+-
  Subtract_a74ec : Sum  Inputs=+-
  Subtract_d1765 : Sum  Inputs=+-
  Subtract_ea8bb : Sum  Inputs=+-
  Blockout_d_psi_gq_SG_D_27_e3839 : Outport
  wires:
  State_psi_gq_SG_D_27_6e8f7/1 -> Add_73542/1
  Constant_x_l_1677c/1 -> Product_3603a/2
  Constant_x_l_d0309/1 -> Product_450c3/2
  Constant_-1_9d686/1 -> Product_57164/1
  Product_57164/1 -> Add_85f35/1
  Constant_x_l_793c4/1 -> Product_57164/2
  Constant_x_l_f9961/1 -> Product_26390/2
  Divide_e205d/1 -> Blockout_d_psi_gq_SG_D_27_e3839/1
  Constant_x_qd_e9e12/1 -> Subtract_d1765/1
  Constant_x_qdd_fe73c/1 -> Add_85f35/2
  Add_e5e6a/1 -> Divide_a909f/2
  Product_fec86/1 -> Divide_638f3/1
  Constant_-1_058df/1 -> Product_3603a/1
  Constant_x_qdd_51bb0/1 -> Subtract_d1765/2
  Constant_x_l_8c285/1 -> Product_9be87/2
  Constant_-1_14efb/1 -> Product_994b8/1
  Constant_x_l_a146c/1 -> Product_994b8/2
  Constant_x_l_54f9f/1 -> Product_56ad6/2
  State_psi_gq_SG_D_27_3e2b9/1 -> Product_c97cd/1
  Add_85f35/1 -> Product_c97cd/2
  Constant_x_qdd_6ad97/1 -> Subtract_2a6c1/2
  Subtract_3ad86/1 -> Product_b10ae/2
  Product_3603a/1 -> Add_c9cb5/1
  Constant_x_qd_20e3c/1 -> Add_c9cb5/2
  Subtract_2a6c1/1 -> Product_8ca79/2
  Constant_x_qd_38946/1 -> Subtract_2a6c1/1
  State_psi_kq_SG_D_27_4dbff/1 -> Product_996e2/1
  Subtract_d1765/1 -> Product_996e2/2
  Product_994b8/1 -> Add_9c560/1
  Add_1e70e/1 -> Product_c8340/2
  Constant_x_qd_d4f0d/1 -> Add_9c560/2
  Product_c97cd/1 -> Divide_b7c1d/1
  Add_c9cb5/1 -> Divide_b7c1d/2
  Product_996e2/1 -> Divide_2b076/1
  Add_9c560/1 -> Divide_2b076/2
  Product_242e9/1 -> Add_7e406/1
  Constant_-1_28226/1 -> Product_242e9/1
  Constant_x_qd_b7f1f/1 -> Add_e5e6a/2
  Constant_x_l_14cc6/1 -> Product_242e9/2
  Constant_x_qdd_699cd/1 -> Subtract_a74ec/2
  Divide_b7c1d/1 -> Subtract_a1eb2/1
  Divide_2b076/1 -> Subtract_a1eb2/2
  Product_9be87/1 -> Add_1e70e/1
  State_psi_q_SG_D_27_a0060/1 -> Add_bba7d/2
  Constant_-1_6b263/1 -> Product_9be87/1
  Constant_x_qd_07190/1 -> Add_7e406/2
  Product_a6325/1 -> Add_c43b7/1
  Constant_x_qd_c908f/1 -> Add_48da1/2
  Subtract_a1eb2/1 -> Add_bba7d/1
  Constant_x_qdd_bfc03/1 -> Add_1e70e/2
  Constant_-1_0983a/1 -> Product_1d788/1
  Product_56ad6/1 -> Add_48da1/1
  Constant_-1_4fa86/1 -> Product_56ad6/1
  Product_450c3/1 -> Add_e5e6a/1
  Add_7e406/1 -> Product_fec86/1
  Constant_-1_3ef3e/1 -> Product_450c3/1
  Add_bba7d/1 -> Product_fec86/2
  Product_c8340/1 -> Divide_cbeb0/1
  State_psi_gq_SG_D_27_ed82f/1 -> Product_c8340/1
  Product_8ca79/1 -> Divide_a909f/1
  State_psi_kq_SG_D_27_09d28/1 -> Product_8ca79/1
  Constant_x_qd_e9b47/1 -> Subtract_a74ec/1
  State_psi_kq_SG_D_27_7c836/1 -> Add_73542/2
  Constant_x_qdd_81391/1 -> Divide_638f3/2
  Constant_-1_14dd2/1 -> Product_26390/1
  Add_48da1/1 -> Divide_cbeb0/2
  Subtract_a74ec/1 -> Product_1d788/2
  Add_73542/1 -> Subtract_ea8bb/1
  Divide_638f3/1 -> Subtract_ea8bb/2
  Product_26390/1 -> Add_b110a/1
  Constant_x_qd_5e3be/1 -> Add_b110a/2
  Divide_cbeb0/1 -> Subtract_808bf/1
  State_psi_q_SG_D_27_f7919/1 -> Add_4b738/2
  Divide_a909f/1 -> Subtract_808bf/2
  Product_1d788/1 -> Product_bef90/1
  Subtract_ea8bb/1 -> Product_bef90/2
  Add_b110a/1 -> Power_6b5ce/1
  Constant_2.0_312bc/1 -> Power_6b5ce/2
  Subtract_808bf/1 -> Add_4b738/1
  Product_bef90/1 -> Divide_4a76a/1
  Power_6b5ce/1 -> Divide_4a76a/2
  Add_4b738/1 -> Divide_647d7/1
  Constant_x_qdd_e17ca/1 -> Divide_647d7/2
  Constant_x_q_90015/1 -> Subtract_84fe7/1
  Constant_x_qd_b0be0/1 -> Subtract_84fe7/2
  Divide_4a76a/1 -> Subtract_3ad86/1
  Constant_-1_d0f9f/1 -> Product_a6325/1
  Divide_647d7/1 -> Subtract_3ad86/2
  State_psi_gq_SG_D_27_c3af2/1 -> Product_a6325/2
  Subtract_84fe7/1 -> Product_b10ae/1
  Product_b10ae/1 -> Add_c43b7/2
  Add_c43b7/1 -> Divide_e205d/1
  Constant_T_qd_feea3/1 -> Divide_e205d/2

== system IEEE30_case/SG_D_27/d_psi_kq_SG_D_27_block ==
  note: d_psi_kq_SG_D_27 in IEEE30_case
      | $-\frac{\psi _{\mathrm{gq},\mathrm{SG},D,27}+\psi _{\mathrm{kq},\mathrm{SG},D,27}+\frac{\left(x_{l}-x_{\mathrm{qd}}\right)\,\left(\psi _{q,\mathrm{SG},D,27}+\frac{\psi _{\mathrm{gq},\mathrm{SG},D,27}\,\left(x_{l}-x_{\mathrm{qdd}}\right)}{x_{l}-x_{\mathrm{qd}}}+\frac{\psi _{\mathrm{kq},\mathrm{SG},D,27}\,\left(x_{\mathrm{qd}}-x_{\mathrm{qdd}}\right)}{x_{l}-x_{\mathrm{qd}}}\right)}{x_{\mathrm{qdd}}}}{T_{\mathrm{qdd}}}$
      | Automatically generated on 2025-11-01 18:38:27 .
  State_psi_gq_SG_D_27_3d919 : Inport
  State_psi_kq_SG_D_27_bbdd7 : Inport  Port=2
  State_psi_gq_SG_D_27_ed697 : Inport  Port=3
  State_psi_kq_SG_D_27_59b97 : Inport  Port=4
  State_psi_q_SG_D_27_76fbd : Inport  Port=5
  Add_14fef : Sum
  Add_292f7 : Sum
  Add_425f6 : Sum
  Add_5229e : Sum
  Add_9711f : Sum
  Add_a8084 : Sum
  Constant_-1_20c8e : Constant  Value=-1
  Constant_-1_36108 : Constant  Value=-1
  Constant_-1_7bbbf : Constant  Value=-1
  Constant_-1_8b8b0 : Constant  Value=-1
  Constant_-1_91c90 : Constant  Value=-1
  Constant_T_qdd_fb9f9 : Constant  Value=T_qdd
  Constant_x_l_52145 : Constant  Value=x_l
  Constant_x_l_68933 : Constant  Value=x_l
  Constant_x_l_90791 : Constant  Value=x_l
  Constant_x_l_df150 : Constant  Value=x_l
  Constant_x_qd_40a14 : Constant  Value=x_qd
  Constant_x_qd_96ab1 : Constant  Value=x_qd
  Constant_x_qd_f07a7 : Constant  Value=x_qd
  Constant_x_qd_f2067 : Constant  Value=x_qd
  Constant_x_qdd_2c0dc : Constant  Value=x_qdd
  Constant_x_qdd_537fe : Constant  Value=x_qdd
  Constant_x_qdd_65a3a : Constant  Value=x_qdd
  Divide_15944 : Product  Inputs=*/
  Divide_4e056 : Product  Inputs=*/
  Divide_9c1f9 : Product  Inputs=*/
  Divide_a3391 : Product  Inputs=*/
  Product_0ab31 : Product
  Product_3b7bd : Product
  Product_45e07 : Product
  Product_56fcf : Product
  Product_64269 : Product
  Product_829eb : Product
  Product_f733b : Product
  Product_f76b7 : Product
  Subtract_1f12a : Sum  Inputs=+-
  Subtract_80892 : Sum  Inputs=+-
  Subtract_c4626 : Sum  Inputs=+-
  Blockout_d_psi_kq_SG_D_27_1e68d : Outport
  wires:
  Constant_-1_8b8b0/1 -> Product_3b7bd/1
  Product_f76b7/1 -> Subtract_80892/1
  Add_5229e/1 -> Product_56fcf/2
  Constant_x_qd_40a14/1 -> Add_14fef/2
  Constant_x_l_90791/1 -> Product_3b7bd/2
  Constant_x_qd_f2067/1 -> Subtract_1f12a/1
  Divide_9c1f9/1 -> Subtract_c4626/1
  Constant_x_l_68933/1 -> Product_0ab31/2
  Product_3b7bd/1 -> Add_425f6/1
  Constant_x_qdd_2c0dc/1 -> Add_425f6/2
  Constant_-1_36108/1 -> Product_0ab31/1
  Add_9711f/1 -> Divide_9c1f9/2
  Constant_x_qdd_537fe/1 -> Subtract_1f12a/2
  Constant_-1_20c8e/1 -> Product_64269/1
  Constant_-1_7bbbf/1 -> Product_829eb/1
  Constant_x_l_df150/1 -> Product_829eb/2
  State_psi_gq_SG_D_27_ed697/1 -> Product_f733b/1
  Add_425f6/1 -> Product_f733b/2
  Divide_15944/1 -> Blockout_d_psi_kq_SG_D_27_1e68d/1
  Add_a8084/1 -> Divide_15944/1
  Product_0ab31/1 -> Add_9711f/1
  Constant_x_qd_f07a7/1 -> Add_9711f/2
  State_psi_kq_SG_D_27_59b97/1 -> Product_45e07/1
  Subtract_1f12a/1 -> Product_45e07/2
  Product_829eb/1 -> Add_14fef/1
  Product_f733b/1 -> Divide_9c1f9/1
  Constant_-1_91c90/1 -> Product_f76b7/1
  Product_45e07/1 -> Divide_a3391/1
  State_psi_kq_SG_D_27_bbdd7/1 -> Subtract_80892/2
  Add_14fef/1 -> Divide_a3391/2
  Constant_x_qdd_65a3a/1 -> Divide_4e056/2
  Constant_x_l_52145/1 -> Product_64269/2
  Divide_a3391/1 -> Subtract_c4626/2
  Product_64269/1 -> Add_292f7/1
  Constant_x_qd_96ab1/1 -> Add_292f7/2
  Subtract_c4626/1 -> Add_5229e/1
  State_psi_q_SG_D_27_76fbd/1 -> Add_5229e/2
  State_psi_gq_SG_D_27_3d919/1 -> Product_f76b7/2
  Add_292f7/1 -> Product_56fcf/1
  Product_56fcf/1 -> Divide_4e056/1
  Subtract_80892/1 -> Add_a8084/1
  Divide_4e056/1 -> Add_a8084/2
  Constant_T_qdd_fb9f9/1 -> Divide_15944/2

== system IEEE30_case/SG_D_27/d_psi_q_SG_D_27_block ==
  note: d_psi_q_SG_D_27 in IEEE30_case
      | $2\,\pi \,f_{0}\,\left(v_{d,\mathrm{SG},D,27}\,\cos\left(\theta _{\mathrm{SG},D,27}\right)+v_{q,\mathrm{SG},D,27}\,\sin\left(\theta _{\mathrm{SG},D,27}\right)-\frac{R_{a}\,\left(\psi _{q,\mathrm{SG},D,27}+\frac{\psi _{\mathrm{gq},\mathrm{SG},D,27}\,\left(x_{l}-x_{\mathrm{qdd}}\right)}{x_{l}-x_{\mathrm{qd}}}+\frac{\psi _{\mathrm{kq},\mathrm{SG},D,27}\,\left(x_{\mathrm{qd}}-x_{\mathrm{qdd}}\right)}{x_{l}-x_{\mathrm{qd}}}\right)}{x_{\mathrm{qdd}}}-\frac{\psi _{d,\mathrm{SG},D,27}\,w_{\mathrm{SG},D,27}}{2\,f_{0}\,\pi }\right)$
      | Automatically generated on 2025-11-01 18:38:10 .
  State_psi_gq_SG_D_27_e40b4 : Inport
  State_psi_kq_SG_D_27_de047 : Inport  Port=2
  State_psi_q_SG_D_27_3920f : Inport  Port=3
  Input_v_d_SG_D_27_8244b : Inport  Port=4
  State_theta_SG_D_27_7e859 : Inport  Port=5
  Input_v_q_SG_D_27_5a914 : Inport  Port=6
  State_theta_SG_D_27_d8fdd : Inport  Port=7
  State_psi_d_SG_D_27_cb123 : Inport  Port=8
  State_w_SG_D_27_1f9a9 : Inport  Port=9
  Add_569a3 : Sum
  Add_71f62 : Sum
  Add_b6e15 : Sum
  Add_e7bb5 : Sum
  Add_f29c5 : Sum
  Constant_-1_11233 : Constant  Value=-1
  Constant_-1_35023 : Constant  Value=-1
  Constant_-1_ca655 : Constant  Value=-1
  Constant_-2.0_c56db : Constant  Value=-2.0
  Constant_2.0_eb10a : Constant  Value=2.0
  Constant_R_a_f01f1 : Constant  Value=R_a
  Constant_f0_30889 : Constant  Value=f0
  Constant_f0_a2408 : Constant  Value=f0
  Constant_pi_bb3bf : Constant  Value=pi
  Constant_pi_c2538 : Constant  Value=pi
  Constant_x_l_09068 : Constant  Value=x_l
  Constant_x_l_96927 : Constant  Value=x_l
  Constant_x_l_b2eef : Constant  Value=x_l
  Constant_x_qd_2cb8a : Constant  Value=x_qd
  Constant_x_qd_aa8b1 : Constant  Value=x_qd
  Constant_x_qd_ac402 : Constant  Value=x_qd
  Constant_x_qdd_24e26 : Constant  Value=x_qdd
  Constant_x_qdd_74f86 : Constant  Value=x_qdd
  Constant_x_qdd_96f44 : Constant  Value=x_qdd
  Divide_20940 : Product  Inputs=*/
  Divide_31127 : Product  Inputs=*/
  Divide_78287 : Product  Inputs=*/
  Divide_c0666 : Product  Inputs=*/
  MathFunc_cos_028d1 : Trigonometry  Operator=cos
  MathFunc_sin_f7226 : Trigonometry
  Product_16c93 : Product
  Product_34238 : Product
  Product_36fcb : Product
  Product_38241 : Product
  Product_516d1 : Product
  Product_8b8e7 : Product
  Product_9faba : Product
  Product_a2ce7 : Product
  Product_b27d8 : Product
  Product_cab66 : Product
  Product_ccc18 : Product
  Product_dce6d : Product
  Product_f49e5 : Product
  Product_fbfee : Product
  Subtract_090f0 : Sum  Inputs=+-
  Subtract_2bc97 : Sum  Inputs=+-
  Subtract_4a5fb : Sum  Inputs=+-
  Subtract_fb06d : Sum  Inputs=+-
  Blockout_d_psi_q_SG_D_27_cf824 : Outport
  wires:
  Constant_f0_30889/1 -> Product_516d1/2
  Constant_x_qdd_24e26/1 -> Add_e7bb5/2
  Constant_-1_35023/1 -> Product_dce6d/1
  Product_dce6d/1 -> Add_e7bb5/1
  Subtract_2bc97/1 -> Subtract_4a5fb/1
  Constant_x_l_b2eef/1 -> Product_dce6d/2
  Divide_c0666/1 -> Subtract_2bc97/1
  Product_ccc18/1 -> Add_f29c5/1
  Constant_-1_11233/1 -> Product_ccc18/1
  Subtract_090f0/1 -> Product_f49e5/2
  Constant_x_qd_2cb8a/1 -> Subtract_090f0/1
  Constant_x_l_09068/1 -> Product_ccc18/2
  Constant_-2.0_c56db/1 -> Product_8b8e7/1
  Constant_x_qdd_96f44/1 -> Subtract_090f0/2
  Product_b27d8/1 -> Add_71f62/1
  Constant_-1_ca655/1 -> Product_b27d8/1
  Constant_x_l_96927/1 -> Product_b27d8/2
  Add_569a3/1 -> Product_a2ce7/2
  Subtract_4a5fb/1 -> Add_569a3/1
  Product_fbfee/1 -> Divide_78287/1
  State_psi_gq_SG_D_27_e40b4/1 -> Product_fbfee/1
  Add_e7bb5/1 -> Product_fbfee/2
  Constant_x_qd_aa8b1/1 -> Add_f29c5/2
  Product_f49e5/1 -> Divide_20940/1
  State_psi_kq_SG_D_27_de047/1 -> Product_f49e5/1
  Constant_x_qd_ac402/1 -> Add_71f62/2
  Add_f29c5/1 -> Divide_78287/2
  Add_71f62/1 -> Divide_20940/2
  Divide_78287/1 -> Subtract_fb06d/1
  Divide_20940/1 -> Subtract_fb06d/2
  Subtract_fb06d/1 -> Add_b6e15/1
  Product_cab66/1 -> Product_9faba/1
  Constant_2.0_eb10a/1 -> Product_cab66/1
  State_psi_q_SG_D_27_3920f/1 -> Add_b6e15/2
  Product_516d1/1 -> Product_a2ce7/1
  Divide_31127/1 -> Add_569a3/2
  Constant_R_a_f01f1/1 -> Product_34238/1
  Add_b6e15/1 -> Product_34238/2
  State_theta_SG_D_27_7e859/1 -> MathFunc_cos_028d1/1
  Product_a2ce7/1 -> Blockout_d_psi_q_SG_D_27_cf824/1
  Constant_pi_c2538/1 -> Product_cab66/2
  Product_34238/1 -> Divide_c0666/1
  Constant_x_qdd_74f86/1 -> Divide_c0666/2
  Input_v_d_SG_D_27_8244b/1 -> Product_36fcb/1
  State_w_SG_D_27_1f9a9/1 -> Product_16c93/2
  MathFunc_cos_028d1/1 -> Product_36fcb/2
  MathFunc_sin_f7226/1 -> Product_38241/2
  State_theta_SG_D_27_d8fdd/1 -> MathFunc_sin_f7226/1
  Product_36fcb/1 -> Subtract_2bc97/2
  Product_38241/1 -> Subtract_4a5fb/2
  Input_v_q_SG_D_27_5a914/1 -> Product_38241/1
  State_psi_d_SG_D_27_cb123/1 -> Product_16c93/1
  Constant_f0_a2408/1 -> Product_9faba/2
  Constant_pi_bb3bf/1 -> Product_8b8e7/2
  Product_16c93/1 -> Divide_31127/1
  Product_8b8e7/1 -> Product_516d1/1
  Product_9faba/1 -> Divide_31127/2

== system IEEE30_case/SG_D_27/d_theta_SG_D_27_block ==
  note: d_theta_SG_D_27 in IEEE30_case
      | $w_{\mathrm{SG},D,27}-2\,\pi \,f_{0}$
      | Automatically generated on 2025-11-01 18:38:34 .
  State_w_SG_D_27_a39e4 : Inport
  Add_e4473 : Sum
  Constant_-2.0_2826d : Constant  Value=-2.0
  Constant_f0_246bb : Constant  Value=f0
  Constant_pi_6ecf5 : Constant  Value=pi
  Product_8c7a4 : Product
  Product_9ea28 : Product
  Blockout_d_theta_SG_D_27_c4116 : Outport
  wires:
  Constant_-2.0_2826d/1 -> Product_9ea28/1
  Product_8c7a4/1 -> Add_e4473/1
  Constant_pi_6ecf5/1 -> Product_9ea28/2
  Product_9ea28/1 -> Product_8c7a4/1
  Constant_f0_246bb/1 -> Product_8c7a4/2
  State_w_SG_D_27_a39e4/1 -> Add_e4473/2
  Add_e4473/1 -> Blockout_d_theta_SG_D_27_c4116/1
